simulink model "subsistema_electrico_corriente_I0s"  (R2023b)
settings: Solver=VariableStepAuto  StartTime=0.0  StopTime=10.0  RelTol=1e-3
InitFcn:
  | parametros
values from neighbouring files (symbols this model uses):
  P_p = 3    [diagrama_polos_y_ceros_LTI.m]    (also in main.m; parametros.m; variacion_de_parametros.m)
settings Model: Creator=Julya  LastModifiedBy=Julya

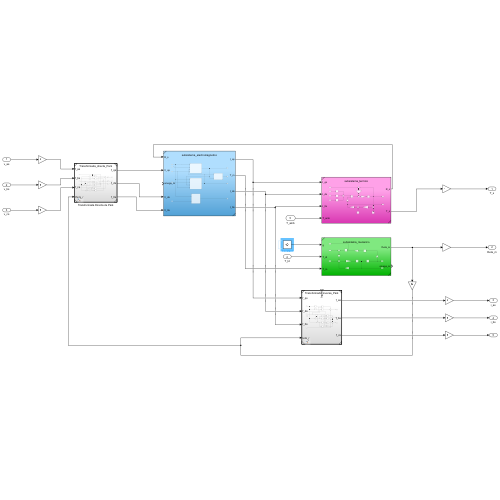
[thumbnail: Simulink's stored preview of the top-level diagram]
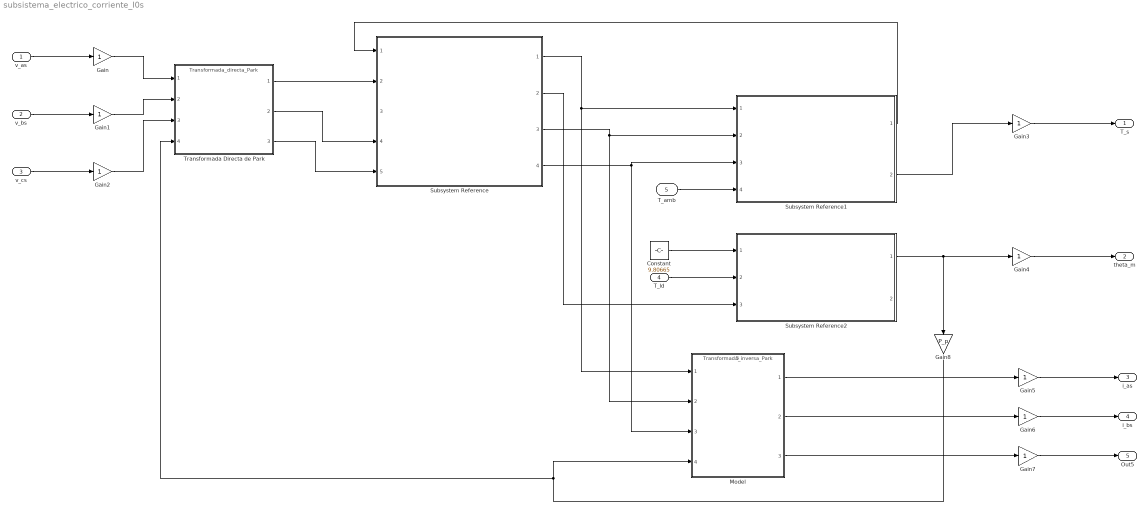
== system subsistema_electrico_corriente_I0s ==
  v_as : Inport
  v_bs : Inport  Port=2
  v_cs : Inport  Port=3
  T_ld : Inport  Port=4
  T_amb : Inport  Port=5
  Constant : Constant  Value=9.80665
  Gain{,1..7} (8 alike) : Gain
  Gain8 : Gain  Gain=P_p
  Model : ModelReference  ModelNameDialog=Transformada_inversa_Park.slx  SimulationMode=Normal  ModelReferenceVersion=1.2
      settings: PortSchema="{\"entries\":[{\"content\":{\"sides\":[{\"content\":{\"connectorIds\":[\"In1\",\"In2\",\"In3\",\"In4\"]},\"type\":\"ConnectorPlacement.EquallySpacedRectSide\",\"uuid\":\"76f5b6d8-1744-47e5-b435-5c8f00b28cfd\"},{\"content\":{\"connectorIds\":[\"Out1\",\"Out2\",\"Out3\"],\"side\":\"RIGHT\"},\"type\":\"ConnectorPlacement.EquallySpacedRectSide\",\"uuid\":\"9de5a2f4-d340-49bc-9846-ef308e173535\"},{\"content\":{\"connectorIds\":[\"In5\"],\"side\":\"TOP\"},\"type\":\"ConnectorPlacement.EquallySpacedRectSide\",\"uuid\":\"ef0b2bb9-d3be-44dc-be3f-e3b27df6b54c\"}]},\"type\":\"ConnectorPlacement.EquallySpacedConnector\",\"uuid\":\"38c54b44-91c8-4fc9-a3d2-29411137fffa\"}],\"packageUris\":[\"http://schema.mathworks.com/mf0/Connector/R2020b\"],\"version\":\"1.0\"}"
  Subsystem Reference : Subsystem  ReferencedSubsystem=subsistema_electromagnetico
  Subsystem Reference1 : Subsystem  ReferencedSubsystem=subsistema_termico
  Subsystem Reference2 : Subsystem  ReferencedSubsystem=subsistema_mecanico
  Transformada Directa de Park : ModelReference  ModelNameDialog=Transformada_directa_Park.slx  SimulationMode=Normal  ModelReferenceVersion=1.2
  T_s : Outport
  theta_m : Outport  Port=2
  i_as : Outport  Port=3
  i_bs : Outport  Port=4
  Out5 : Outport  Port=5
  wires:
  Transformada Directa de Park/1 -> Subsystem Reference/2
  Transformada Directa de Park/2 -> Subsystem Reference/4
  Transformada Directa de Park/3 -> Subsystem Reference/5
  Subsystem Reference/1 -> Model/1, Subsystem Reference1/1
  Subsystem Reference/3 -> Model/2, Subsystem Reference1/2
  Subsystem Reference/4 -> Subsystem Reference1/3, Model/3
  Subsystem Reference1/1 -> Subsystem Reference/1
  Subsystem Reference1/2 -> Gain3/1
  Gain3/1 -> T_s/1
  Subsystem Reference2/1 -> Gain8/1, Gain4/1
  Gain4/1 -> theta_m/1
  Subsystem Reference/2 -> Subsystem Reference2/3
  T_ld/1 -> Subsystem Reference2/2
  Gain5/1 -> i_as/1
  Gain6/1 -> i_bs/1
  Gain7/1 -> Out5/1
  v_as/1 -> Gain/1
  v_bs/1 -> Gain1/1
  v_cs/1 -> Gain2/1
  Gain/1 -> Transformada Directa de Park/1
  Gain1/1 -> Transformada Directa de Park/2
  Gain2/1 -> Transformada Directa de Park/3
  Gain8/1 -> Transformada Directa de Park/4, Model/4
  Model/3 -> Gain7/1
  Model/2 -> Gain6/1
  Model/1 -> Gain5/1
  T_amb/1 -> Subsystem Reference1/4
  Constant/1 -> Subsystem Reference2/1
